simulink model "plasmaless_timestep"  (R2022a)
settings: Solver=FixedStepAuto  StartTime=0.0  StopTime=10.0  RelTol=1e-3
values from neighbouring files (symbols this model uses):
  A = sysd_plasmaless.A    [configure_plasmaless_model.m]    (also in timeseries_plasmaless_model.m = 10)
  B = sysd_plasmaless.B    [configure_plasmaless_model.m]
  C = sysd_plasmaless.C    [configure_plasmaless_model.m]
  D = sysd_plasmaless.D    [configure_plasmaless_model.m]
  x0 = zeros(size(A,1),1)    [run_plasmaless_model.m]
settings Model: Creator=pesamof  LastModifiedBy=pesamof

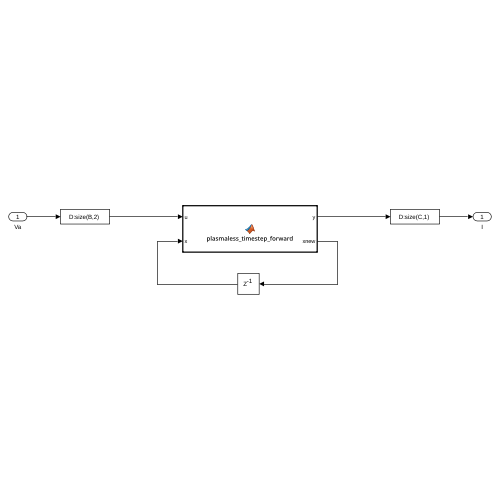
[thumbnail: Simulink's stored preview of the top-level diagram]
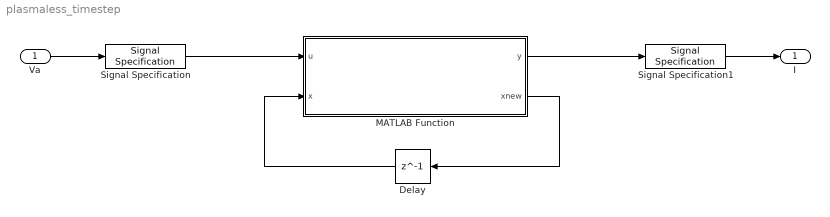
== system plasmaless_timestep ==
  Va : Inport
  Delay : Delay  DelayLength=1  InitialCondition=x0
  MATLAB Function : MATLAB Function  TreatAsAtomicUnit=on
  Signal Specification : SignalSpecification  Dimensions=size(B,2)
  Signal Specification1 : SignalSpecification  Dimensions=size(C,1)
  I : Outport
  wires:
  MATLAB Function/2(xnew) -> Delay/1
  Delay/1 -> MATLAB Function/2(x)
  MATLAB Function/1(y) -> Signal Specification1/1
  Va/1 -> Signal Specification/1
  Signal Specification/1 -> MATLAB Function/1(u)
  Signal Specification1/1 -> I/1

== matlab function plasmaless_timestep/MATLAB Function ==
  data: u input; y output; x input; xnew output; A parameter; B parameter; C parameter; D parameter
function [y,xnew] = plasmaless_timestep_forward(u,x,A,B,C,D)
% evolve state space model for plasmaless electromagnetic dynamics

xnew = A*x + B*u;
y = C*x + D*u;
